simulink model "adm_pcie_9h7_dts_dual_4x100g_dts_test"  (R2019a)
settings: Solver=VariableStepAuto  StartTime=0.0  StopTime=10.0  RelTol=1e-3
undefined symbols (not defined in the file or in its folder): datetime, posixtime
libraries: xbsIndex_r4 x4914, casper_library_misc x38, xps_library x11
(part 1 of 58)
settings Model: ModifiedComment=jackh -- Wed Aug 24 09:07:48 2022 -- Version 1.233  Creator=jackh  LastModifiedBy=jackh
settings Model: ModifiedHistory=|
  | jackh -- Wed Aug 24 09:07:48 2022 -- Version 1.233
  | 
  | jackh -- Tue Aug 23 10:15:12 2022 -- Version 1.232
  | 
  | jackh -- Tue Aug 23 10:08:31 2022 -- Version 1.231
  | 
  | jackh -- Thu Aug 18 20:38:32 2022 -- Version 1.230
  | 
  | v13.4 bugfix 1
  | Rebuild with DTS buffer fixes
  | 
  | jackh -- Thu Aug 04 11:53:58 2022 -- Version 1.229
  | 
  | as compiled
  | 
  | jackh -- Wed Aug 03 18:39:00 2022 -- Version 1.228
  | 
  | v13.4 -- add post quant TVG which is a counter with spectrum number
  | 
  | jackh -- Wed Aug 03 12:22:54 2022 -- Version 1.227
  | 
  | as compiled
  | 
  | jackh -- Tue Aug 02 16:59:19 2022 -- Version 1.226
  | 
  | v13.3.3
  | 
  | Make LO offset input accept signed values
  | 
  | jackh -- Thu Jul 14 12:25:27 2022 -- Version 1.225
  | v13.3.2
  | 
  | change sine/cos lookup tables to 18-bit depth
  | 
  | jackh -- Fri Jul 08 12:09:48 2022 -- Version 1.224
  | 
  | jackh -- Fri Jul 08 11:59:21 2022 -- Version 1.223
  | 
  | 13.3.1
  | 
  | Make LO shift phase register 32_29
  | 
  | jackh -- Tue Jul 05 14:22:39 2022 -- Version 1.222
  | 
  | 13.2.4
  | 
  | Add 100G output snapshots and stats counters
  | 
  | jackh -- Fri Jun 17 09:21:46 2022 -- Version 1.221
  | 
  | Make PR template file relative. Increment fw revision
  | 
  | jackh -- Fri May 20 08:03:37 2022 -- Version 1.220
  | 
  | jackh -- Thu May 19 16:47:03 2022 -- Version 1.219
  | 
  | jackh -- Thu May 19 16:07:36 2022 -- Version 1.218
  | 
  | 13.2.2
  | 
  | Increase coarse delay to 512 samples
  | 
  | jackh -- Thu May 19 15:48:23 2022 -- Version 1.217
  | 
  | pipeline time offset
  | 
  | jackh -- Thu May 19 15:45:17 2022 -- Version 1.216
  | 
  | v13.2.1
  | 
  | Add aux time measurement
  | 
  | jackh -- Tue May 03 22:22:24 2022 -- Version 1.215
  | 
  | jackh -- Tue May 03 12:52:13 2022 -- Version 1.214
  | 
  | 13.2.0.1
  | 
  | - Fix FFT syncout period (now infinite)
  | - Add max_delay register to delay subsystem
  | 
  | jackh -- Tue May 03 11:06:51 2022 -- Version 1.213
  | 
  | v13.2 (should have been 13) as compiled
  | 
  | jackh -- Mon May 02 12:19:53 2022 -- Version 1.212
  | 
  | jackh -- Mon May 02 12:13:43 2022 -- Version 1.211
  | 
  | jackh -- Mon May 02 12:03:22 2022 -- Version 1.210
  | 
  | Move to 1MHz channels (2048-chan PFB; 1024 sent chans)
  | Incorporate FFT descramble mlib_devel fix
  | 
  | jackh -- Thu Apr 07 10:41:20 2022 -- Version 1.209
  | 
  | compiled
  | 
  | jackh -- Wed Apr 06 17:17:38 2022 -- Version 1.208
  | 
  | Bugfix 1
  | 
  | - Change LO offset so real part os cosine mixer (so mixing with DC does nothing)
  | - Fix cross-corr conjugation
  | - Fix cross corr acc_len computation
  | 
  | jackh -- Thu Mar 24 11:16:10 2022 -- Version 1.207
  | 
  | jackh -- Wed Mar 23 15:55:29 2022 -- Version 1.206
  | 
  | v12.2 Add sine wave generators to both pipelines.
  | Default to no added sine wave.
  | 
  | jackh -- Wed Mar 23 15:38:55 2022 -- Version 1.205
  | 
  | jackh -- Wed Mar 23 15:24:07 2022 -- Version 1.204
  | 
  | delay match sine generation and data streams
  | 
  | jackh -- Wed Mar 23 15:22:28 2022 -- Version 1.203
  | 
  | jackh -- Wed Mar 23 15:14:26 2022 -- Version 1.202
  | 
  | Add additive sinewave TVG
  | 
  | jackh -- Wed Mar 23 15:12:01 2022 -- Version 1.201
  | 
  | jackh -- Tue Mar 08 10:23:22 2022 -- Version 1.200
  | 
  | jackh -- Mon Mar 07 17:18:28 2022 -- Version 1.199
  | 
  | jackh -- Mon Mar 07 17:10:55 2022 -- Version 1.198
  | 
  | jackh -- Mon Mar 07 16:45:17 2022 -- Version 1.197
  | 
  | jackh -- Mon Mar 07 16:37:10 2022 -- Version 1.196
  | 
  | Add Corr block.
  | Allows examination of post-quantization signals, and
  | to cross correlate different IFs (useful for testing
  | in internal noisegen mode)
  | 
  | jackh -- Mon Mar 07 16:13:50 2022 -- Version 1.195
  | 
  | PFB band select reorder depth fix
  | 
  | jackh -- Thu Mar 03 13:08:01 2022 -- Version 1.194
  | 
  | jackh -- Tue Mar 01 20:34:16 2022 -- Version 1.193
  | 
  | jackh -- Tue Mar 01 17:19:43 2022 -- Version 1.192
  | 
  | jackh -- Tue Mar 01 17:10:04 2022 -- Version 1.191
  | 
  | jackh -- Tue Mar 01 16:55:54 2022 -- Version 1.190
  | 
  | jackh -- Tue Mar 01 16:45:57 2022 -- Version 1.189
  | 
  | jackh -- Tue Mar 01 15:57:56 2022 -- Version 1.188
  | 
  | jackh -- Tue Mar 01 15:49:45 2022 -- Version 1.187
  | 
  | jackh -- Tue Mar 01 15:22:14 2022 -- Version 1.186
  | 
  | jackh -- Mon Feb 28 13:26:19 2022 -- Version 1.185
  | 
  | jackh -- Mon Feb 28 13:08:19 2022 -- Version 1.184
  | 
  | jackh -- Sat Feb 26 14:41:54 2022 -- Version 1.183
  | 
  | jackh -- Fri Feb 25 18:46:11 2022 -- Version 1.182
  | 
  | jackh -- Fri Feb 25 18:45:03 2022 -- Version 1.181
  | 
  | jackh -- Thu Feb 24 15:51:36 2022 -- Version 1.180
  | 
  | update noisegen casting (just take MSBs)
  | 
  | jackh -- Thu Feb 24 15:08:58 2022 -- Version 1.179
  | 
  | v12
  | 
  | jackh -- Thu Feb 24 15:06:46 2022 -- Version 1.178
  | 
  | Move to 4x100G template
  | 
  | 
  | jackh -- Thu Feb 24 15:02:10 2022 -- Version 1.177
  | 
  | jackh -- Wed Feb 09 19:02:50 2022 -- Version 1.176
  | 
  | jackh -- Wed Feb 09 10:59:16 2022 -- Version 1.175
  | 
  | Try _again_ to fix timestamp issue.
  | This time the fix was actually simulated, and seems to work.
  | 
  | jackh -- Wed Feb 09 10:58:22 2022 -- Version 1.174
  | 
  | jackh -- Wed Feb 09 10:34:47 2022 -- Version 1.173
  | 
  | jackh -- Tue Feb 08 22:13:18 2022 -- Version 1.172
  | 
  | Change autocorr pipelining to fix timing errors
  | 
  | jackh -- Tue Feb 08 11:22:49 2022 -- Version 1.171
  | 
  | Try (again) to fix MCNT offset issue.
  | This time just propagate the time_step_bit lower MCNT counter
  | bits through to the header.
  | 
  | jackh -- Tue Feb 08 08:36:48 2022 -- Version 1.170
  | 
  | jackh -- Mon Feb 07 16:56:49 2022 -- Version 1.169
  | 
  | jackh -- Mon Feb 07 16:34:15 2022 -- Version 1.168
  | 
  | jackh -- Mon Feb 07 16:26:49 2022 -- Version 1.167
  | 
  | jackh -- Mon Feb 07 12:47:03 2022 -- Version 1.166
  | 
  | jackh -- Mon Feb 07 12:32:35 2022 -- Version 1.165
  | 
  | Add TT sync register, storing the time of the last sync
  | 
  | jackh -- Mon Feb 07 12:23:30 2022 -- Version 1.164
  | 
  | increment bugfix to 11.0.0.2
  | 
  | 
  | jackh -- Mon Feb 07 12:22:16 2022 -- Version 1.163
  | 
  | Propagate LSBs of sync time to packet headers
  | 
  | jackh -- Sat Feb 05 22:32:38 2022 -- Version 1.162
  | 
  | jackh -- Sat Feb 05 18:43:37 2022 -- Version 1.161
  | 
  | v11
  | More changes to reorder.
  | Process ADC data at 8 (not 12) bit resolution
  | Use URAM via black-box imports for coarse delay and big channel reorder
  | 
  | jackh -- Sat Feb 05 18:36:04 2022 -- Version 1.160
  | 
  | jackh -- Sat Feb 05 17:38:40 2022 -- Version 1.159
  | 
  | jackh -- Sat Feb 05 17:24:29 2022 -- Version 1.158
  | 
  | jackh -- Sat Feb 05 17:22:21 2022 -- Version 1.157
  | 
  | jackh -- Fri Feb 04 17:40:07 2022 -- Version 1.156
  | 
  | jackh -- Fri Feb 04 12:37:39 2022 -- Version 1.155
  | 
  | 64 times per packet
  | 
  | 
  | jackh -- Thu Feb 03 21:55:46 2022 -- Version 1.154
  | 
  | as compiled
  | 
  | 
  | jackh -- Thu Feb 03 14:45:04 2022 -- Version 1.153
  | 
  | jackh -- Thu Feb 03 14:28:02 2022 -- Version 1.152
  | 
  | jackh -- Thu Feb 03 13:59:18 2022 -- Version 1.151
  | 
  | jackh -- Thu Feb 03 11:15:21 2022 -- Version 1.150
  | 
  | jackh -- Wed Feb 02 16:47:47 2022 -- Version 1.149
  | 
  | jackh -- Wed Feb 02 16:40:11 2022 -- Version 1.148
  | 
  | Fix incorrect final transpose in reorder block
  | 
  | jackh -- Wed Feb 02 16:16:13 2022 -- Version 1.147
  | 
  | v8. Add channel reordering
  | 
  | Not actually necessary for 8-bit mode, but will
  | facilitate testing which is necessary for 3-bit mode
  | 
  | jackh -- Wed Feb 02 10:37:50 2022 -- Version 1.146
  | 
  | 7.0.1
  | 
  | Change coarse delay bram latency to 3 (hopefully will fix small timing fail)
  | 
  | jackh -- Wed Feb 02 10:34:03 2022 -- Version 1.145
  | 
  | jackh -- Tue Feb 01 14:52:02 2022 -- Version 1.144
  | 
  | Don't use ultraRAM for coarse delay (but we should!)
  | because it breaks sysgen. Sigh.
  | 
  | jackh -- Tue Feb 01 14:27:12 2022 -- Version 1.143
  | 
  | jackh -- Tue Feb 01 14:18:24 2022 -- Version 1.142
  | 
  | v7. Add noisegen / coarse delay
  | 
  | jackh -- Tue Feb 01 14:12:26 2022 -- Version 1.141
  | 
  | jackh -- Tue Feb 01 14:09:37 2022 -- Version 1.140
  | 
  | jackh -- Tue Feb 01 11:46:40 2022 -- Version 1.139
  | 
  | jackh -- Tue Feb 01 11:12:13 2022 -- Version 1.138
  | 
  | Add noise gen
  | 
  | jackh -- Tue Feb 01 11:01:17 2022 -- Version 1.137
  | 
  | v6.1 Harmonize input ordering convention by flipping
  | inputs so "input 0" is MSBs of data
  | 
  | jackh -- Tue Feb 01 10:38:57 2022 -- Version 1.136
  | 
  | jackh -- Mon Jan 31 13:11:04 2022 -- Version 1.135
  | 
  | jackh -- Mon Jan 31 12:33:38 2022 -- Version 1.134
  | 
  | jackh -- Mon Jan 31 12:25:15 2022 -- Version 1.133
  | 
  | jackh -- Fri Jan 28 17:22:49 2022 -- Version 1.132
  | 
  | jackh -- Fri Jan 28 17:16:19 2022 -- Version 1.131
  | 
  | jackh -- Fri Jan 28 17:06:25 2022 -- Version 1.130
  | 
  | v6.0 Add input bitstats / simulation mux
  | 
  | jackh -- Fri Jan 28 17:02:52 2022 -- Version 1.129
  | 
  | jackh -- Fri Jan 28 16:59:39 2022 -- Version 1.128
  | 
  | jackh -- Fri Jan 28 16:55:40 2022 -- Version 1.127
  | 
  | jackh -- Fri Jan 28 16:17:24 2022 -- Version 1.126
  | 
  | v5.0.2 Fix potential (but unliekly) issue with sync arm coinciding
  | with sync pulse
  | 
  | 
  | jackh -- Fri Jan 28 16:01:17 2022 -- Version 1.125
  | 
  | Attempt to fix DTS alignment unreliability (control signal CDC issue in mlib_devel)
  | 
  | jackh -- Fri Jan 28 12:51:42 2022 -- Version 1.124
  | 
  | as compiled
  | 
  | jackh -- Thu Jan 27 16:47:33 2022 -- Version 1.123
  | 
  | v5.0
  | 
  | Add sync gen logic
  | 
  | jackh -- Thu Jan 27 11:25:49 2022 -- Version 1.122
  | 
  | v4.1 Add index interval error counter
  | 
  | jackh -- Thu Jan 27 11:22:02 2022 -- Version 1.121
  | 
  | Make index 50ms -- add not-locked counter
  | 
  | 
  | jackh -- Thu Jan 27 10:32:00 2022 -- Version 1.120
  | 
  | Recompile using raw "index" pulse. Add index snapshots
  | 
  | jackh -- Wed Jan 26 15:06:47 2022 -- Version 1.119
  | 
  | jackh -- Wed Jan 26 13:46:28 2022 -- Version 1.118
  | 
  | jackh -- Wed Jan 26 13:04:56 2022 -- Version 1.117
  | 
  | jackh -- Tue Jan 25 18:32:15 2022 -- Version 1.116
  | 
  | Add index (10ms pulse?) count logic
  | 
  | jackh -- Tue Jan 25 18:31:36 2022 -- Version 1.115
  | 
  | jackh -- Tue Jan 25 11:48:12 2022 -- Version 1.114
  | 
  | jackh -- Tue Jan 25 11:41:44 2022 -- Version 1.113
  | 
  | jackh -- Tue Jan 25 11:38:37 2022 -- Version 1.112
  | 
  | Readd autocorr (needed behavioural complex mults)
  | 
  | jackh -- Mon Jan 24 20:49:54 2022 -- Version 1.111
  | 
  | comment out autocorr (causing compile fails)
  | 
  | jackh -- Mon Jan 24 20:10:36 2022 -- Version 1.110
  | 
  | jackh -- Mon Jan 24 19:58:33 2022 -- Version 1.109
  | 
  | jackh -- Mon Jan 24 19:53:28 2022 -- Version 1.108
  | 
  | autocorr floating point error fixes
  | 
  | 
  | jackh -- Mon Jan 24 19:51:34 2022 -- Version 1.107
  | 
  | jackh -- Mon Jan 24 18:28:31 2022 -- Version 1.106
  | 
  | jackh -- Mon Jan 24 18:27:12 2022 -- Version 1.105
  | 
  | Add autocorr (to pipeline 0)
  | 
  | jackh -- Mon Jan 24 18:15:24 2022 -- Version 1.104
  | 
  | Add EQTVG
  | 
  | jackh -- Mon Jan 24 13:19:54 2022 -- Version 1.103
settings DataIOCC: ReturnWorkspaceOutputs=off
settings DebuggingCC: PregeneratedLibrarySubsystemCodeDiagnostic=none  ArithmeticOperatorsInVariantConditions=warning
settings SFSimCC: SimUseLocalCustomCode=off
settings RTWCC: RTWUseLocalCustomCode=off

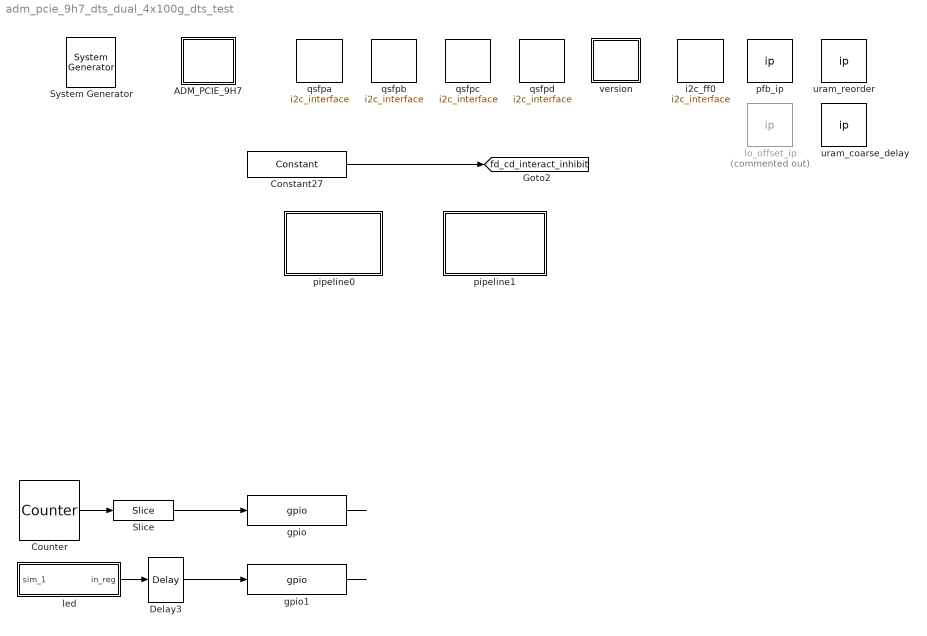
== system adm_pcie_9h7_dts_dual_4x100g_dts_test ==
  " System Generator" : xbsIndex_r4/ System Generator  Tag=genX  xilinxfamily=virtexuplusHBM  part=xcvu37p  speed=-2-e  package=fsvh2892  synthesis_tool=XST  clock_wrapper=Clock Enables  directory=/home/jackh/src/vla-dev/firmware/adm_pcie_9h7_dts_dual_4x100g_dts_test/sysgen  proj_type=Vivado  Synth_file=Vivado Synthesis Defaults  Impl_file=Vivado Implementation Defaults  testbench=off  simulink_period=1  sysclk_period=3.9062  dcm_input_clock_period=10  incr_netlist=off  trim_vbits=Everywhere in SubSystem  dbl_ovrd=According to Block Masks  core_generation=According to Block Masks  run_coregen=off  deprecated_control=off  eval_field=0  block_type=sysgen
  ADM_PCIE_9H7 : Subsystem  Tag=xps:xsg  mask(xsg core config){hw_sys=ADM_PCIE_9H7:xcvu37p, clk_src=dts_clk, clk_rate=256, use_microblaze=off, use_pr=on, pr_template=[fileparts(which(bdroot)) '/pr_templates/adm_pcie_9h7_dts_dual_4x100g_pr_template-no-ip.xpr.zip'], sample_period=1, synthesis_tool=XST}
      mask prompts: hw_sys "Hardware Platform"; clk_src "User IP Clock source"; clk_rate "User IP Clock Rate (MHz)"; use_microblaze "Use Microblaze controller?"; use_pr "Use PCIe Partial Reconfiguration"; sample_period "Sample Period"; synthesis_tool "Synthesis Tool:"
      mask help:
      | The XSG Core Config block is used to configure the System Generator design
      | for the casper_xps toolflow. Settings here are used to configure the
      | Xilinx System Generator block parameters automatically, and control toolflow
      | script  execution. It needs to be at the top level of all designs being compiled
      | with the casper_xps toolflow.
      mask init:
      | xps_xsg_adm_pcie_9h7_conf_mask;
      mask Help: eval('xlWeb([getenv(''MLIB_ROOT''), ''\doc\html\sys_xsg_core_config\sys_xsg_core_config.html''])')
      mask TypeOptions hw_sys: ADM_PCIE_9H7:xcvu37p
      mask TypeOptions clk_src: sys_clk | dts_clk
      mask TypeOptions synthesis_tool: Leonardo Spectrum | Synplify | Synplify Pro | XST
      mask Display: fprintf(['ADM\nPCIE_9H7']);
  Constant27 : xbsIndex_r4/Constant  const=1  gui_display_data_type=Boolean  arith_type=Boolean  n_bits=32  bin_pt=31  preci_type=Single  exp_width=8  frac_width=24  explicit_period=on  period=1  equ=P=C  opselect=C  inp2=PCIN>>17  opr=+  inp1=P  carry=CIN  dbl_ovrd=off  block_type=constant
  Counter : xbsIndex_r4/Counter  cnt_type=Free Running  cnt_to=Inf  operation=Up  start_count=0  cnt_by_val=1  arith_type=Unsigned  n_bits=27  bin_pt=0  load_pin=off  rst=off  en=off  explicit_period=on  period=1  use_behavioral_HDL=off  implementation=Fabric  dbl_ovrd=off  block_type=counter
  Delay3 : xbsIndex_r4/Delay  rst=off  infoeditControl=Selection of Reset will increase slice count due to use of real FFs and instead of SRLs  en=off  latency=1  reg_retiming=off  dbl_ovrd=off  block_type=delay
  Slice : xbsIndex_r4/Slice  nbits=2  boolean_output=off  mode=Upper Bit Location + Width  bit1=0  base1=MSB of Input  bit0=0  base0=LSB of Input  dbl_ovrd=off  block_type=slice
  gpio : xps_library/IO/gpio  Tag=xps:gpio  io_group_params_forwarded=off  io_group=ROACH:led  io_group_real=led  io_group_custom=0  io_dir=out  arith_type=Unsigned  bitwidth=2  bin_pt=0  bit_index=[0 1]  sample_period=1  use_single_ended=off  use_ddr=off  reg_iob=on  reg_clk_phase=0  termination=None
      settings: SourceProductName=CASPER XPS Blockset
  gpio1 : xps_library/IO/gpio  Tag=xps:gpio  io_group_params_forwarded=off  io_group=ROACH:led  io_group_real=led  io_group_custom=0  io_dir=out  arith_type=Boolean  bitwidth=1  bin_pt=0  bit_index=2  sample_period=1  use_single_ended=off  use_ddr=off  reg_iob=on  reg_clk_phase=0  termination=None
      settings: SourceProductName=CASPER XPS Blockset
  i2c_ff0 : xps_library/IO/i2c_interface  Tag=xps:i2c_interface  sda_gpio='gpio'  sda_gpio_index=8  scl_gpio='gpio'  scl_gpio_index=7
      settings: SourceProductName=CASPER XPS Blockset
  led : Subsystem  Tag=xps:sw_reg  AncestorBlock=xps_library/Memory/software_register  mask(swreg){io_dir=From Processor, io_delay=0, init_val=0, sample_period=1, names=reg, bitwidths=1, bin_pts=0, arith_types=2, sim_port=on, show_format=on}
      mask prompts: io_dir "I/O direction"; io_delay "I/O delay"; init_val "Initial Value"; sample_period "Sample period"; names "Bitfield names [msb...lsb]"; bitwidths "Bitfield widths"; bin_pts "Bitfield binary pts"; arith_types "Bitfield types, ufix=0, fix=1, bool=2"; sim_port "Provide sim input/output?"; show_format "Print format string?"
      mask help: A 32-bit software-accessible register. Can be divided into bitfields of varying widths and types using the fields in the block mask.
      mask init:
      | swreg_init(gcb)
      settings: AttributesFormatString=1input:b = 1 bits
      mask TypeOptions io_dir: To Processor | From Processor
      mask Callback io_dir:
      | mask_enables = get_param(gcb, 'MaskEnables');
      | mask_names = get_param(gcb, 'MaskNames');
      | if strcmp(get_param(gcb, 'io_dir'), 'To Processor'),
      |     mask_enables{ismember(mask_names, 'sample_period')} = 'off';
      | else
      |     mask_enables{ismember(mask_names, 'sample_period')} = 'on';
      | end
      | set_param(gcb, 'MaskEnables', mask_enables);
      mask DialogControl ParameterTabVar0 Prompt: Setup
  lo_offset_ip : xps_library/Utilities/ip  Tag=xps:ip  Commented=on  lib_path=[fileparts(which(bdroot)) '/dsp/mixer_dec_8x_8i_8o_core']  ip_name='mixer_dec_8x_8i_8o_core'
      settings: SourceProductName=CASPER XPS Blockset
  pfb_ip : xps_library/Utilities/ip  Tag=xps:ip  lib_path=[fileparts(which(bdroot)) '/dsp/pfb_cplx_2p_2048c_16i_18o_core']  ip_name='pfb_cplx_2p_2048c_16i_18o_core'
      settings: SourceProductName=CASPER XPS Blockset
  pipeline0 : Subsystem
  pipeline1 : Subsystem
  qsfpa : xps_library/IO/i2c_interface  Tag=xps:i2c_interface  sda_gpio='qsfp_sda'  sda_gpio_index=0  scl_gpio='qsfp_scl'  scl_gpio_index=0
      settings: SourceProductName=CASPER XPS Blockset
  qsfpb : xps_library/IO/i2c_interface  Tag=xps:i2c_interface  sda_gpio='qsfp_sda'  sda_gpio_index=1  scl_gpio='qsfp_scl'  scl_gpio_index=1
      settings: SourceProductName=CASPER XPS Blockset
  qsfpc : xps_library/IO/i2c_interface  Tag=xps:i2c_interface  sda_gpio='qsfp_sda'  sda_gpio_index=2  scl_gpio='qsfp_scl'  scl_gpio_index=2
      settings: SourceProductName=CASPER XPS Blockset
  qsfpd : xps_library/IO/i2c_interface  Tag=xps:i2c_interface  sda_gpio='qsfp_sda'  sda_gpio_index=3  scl_gpio='qsfp_scl'  scl_gpio_index=3
      settings: SourceProductName=CASPER XPS Blockset
  uram_coarse_delay : xps_library/Utilities/ip  Tag=xps:ip  lib_path=[fileparts(which(bdroot)) '/dsp/uram_dp_64kx64_latency3_core']  ip_name='uram_dp_64kx64_latency3_core'
      settings: SourceProductName=CASPER XPS Blockset
  uram_reorder : xps_library/Utilities/ip  Tag=xps:ip  lib_path=[fileparts(which(bdroot)) '/dsp/uram_8192x512_latency3_core']  ip_name='uram_8192x512_latency3_core'
      settings: SourceProductName=CASPER XPS Blockset
  version : Subsystem  mask{fw_type=99, ver_maj=1, ver_min=0, ver_rev=0, ver_bugfix=0}
      mask prompts: fw_type "Firmware Type"; ver_maj "Major version"; ver_min "Minor version"; ver_rev "Revision"; ver_bugfix "Bugfix"
  tag scope: fd_cd_interact_inhibit=global
  wires:
  gpio/1 -> ?
  Delay3/1 -> gpio1/1
  Counter/1 -> Slice/1
  gpio1/1 -> ?
  led/1(in_reg) -> Delay3/1
  Slice/1 -> gpio/1
  Constant27/1 -> [fd_cd_interact_inhibit]

== system adm_pcie_9h7_dts_dual_4x100g_dts_test/ADM_PCIE_9H7 ==

== system adm_pcie_9h7_dts_dual_4x100g_dts_test/led ==
  sim_1 : Inport
  adm_pcie_9h7_dts_dual_4x100g_dts_test_led_user_data_out : xbsIndex_r4/Gateway In  gui_display_data_type=Fixed-point  arith_type=Unsigned  n_bits=32  bin_pt=0  preci_type=Single  exp_width=8  frac_width=24  rows=1  columns=1  quantization="Round  (unbiased: +/- Inf)"  overflow=Saturate  period=1  UseAsADC=off  ADCChannel='1'  interface=None  automatic_assignment=on  address_offset=hex2dec('00')  intf_name=''  intf_description=''  default_value=0  timing_constraint=None  locs_specified=off  LOCs={}  io_standard={}  inherit_from_input=off  hdl_port=on  dbl_ovrd=off  block_type=gatewayin
  convert1_1 : DataTypeConversion  OutDataTypeStr=fixdt('ufix1_En0')  LockScale=on
  convert2_1 : DataTypeConversion  OutDataTypeStr=fixdt('ufix1_En0')  ConvertRealWorld=Stored Integer (SI)  LockScale=on
  gain_1 : Gain
  io_delay : xbsIndex_r4/Delay  rst=off  infoeditControl=Selection of Reset will increase slice count due to use of real FFs and instead of SRLs  en=off  latency=0  reg_retiming=on  dbl_ovrd=off  block_type=delay
  slice_reg : xbsIndex_r4/Slice  nbits=1  boolean_output=on  mode=Lower Bit Location + Width  bit1=0  base1=MSB of Input  bit0=0  base0=LSB of Input  dbl_ovrd=off  block_type=slice
  in_reg : Outport
  wires:
  adm_pcie_9h7_dts_dual_4x100g_dts_test_led_user_data_out/1 -> io_delay/1
  sim_1/1 -> convert1_1/1
  convert1_1/1 -> convert2_1/1
  convert2_1/1 -> gain_1/1
  gain_1/1 -> adm_pcie_9h7_dts_dual_4x100g_dts_test_led_user_data_out/1
  io_delay/1 -> slice_reg/1
  slice_reg/1 -> in_reg/1

== system adm_pcie_9h7_dts_dual_4x100g_dts_test/pipeline0 ==
  note: 4 inputs (2 IFs x dual pol)
      |
      | Each 8 parallel words x 12 bits
      | (96 bits per input)
      | (384 bits total)
  Constant : xbsIndex_r4/Constant  const=0  gui_display_data_type=Fixed-point  arith_type=Unsigned  n_bits=64  bin_pt=0  preci_type=Single  exp_width=8  frac_width=24  explicit_period=on  period=1  equ=P=C  opselect=C  inp2=PCIN>>17  opr=+  inp1=P  carry=CIN  dbl_ovrd=off  block_type=constant
  Constant1 : xbsIndex_r4/Constant  const=0  gui_display_data_type=Fixed-point  arith_type=Unsigned  n_bits=16  bin_pt=0  preci_type=Single  exp_width=8  frac_width=24  explicit_period=on  period=1  equ=P=C  opselect=C  inp2=PCIN>>17  opr=+  inp1=P  carry=CIN  dbl_ovrd=off  block_type=constant
  Constant{3..4,9..10} (4 alike) : xbsIndex_r4/Constant  const=0  gui_display_data_type=Boolean  arith_type=Boolean  n_bits=32  bin_pt=0  preci_type=Single  exp_width=8  frac_width=24  explicit_period=on  period=1  equ=P=C  opselect=C  inp2=PCIN>>17  opr=+  inp1=P  carry=CIN  dbl_ovrd=off  block_type=constant
  Constant11 : xbsIndex_r4/Constant  const=0  gui_display_data_type=Fixed-point  arith_type=Unsigned  n_bits=512  bin_pt=0  preci_type=Single  exp_width=8  frac_width=24  explicit_period=on  period=1  equ=P=C  opselect=C  inp2=PCIN>>17  opr=+  inp1=P  carry=CIN  dbl_ovrd=off  block_type=constant
  Constant2 : xbsIndex_r4/Constant  const=0  gui_display_data_type=Fixed-point  arith_type=Unsigned  n_bits=32  bin_pt=0  preci_type=Single  exp_width=8  frac_width=24  explicit_period=on  period=1  equ=P=C  opselect=C  inp2=PCIN>>17  opr=+  inp1=P  carry=CIN  dbl_ovrd=off  block_type=constant
  Constant5 : xbsIndex_r4/Constant  const=0  gui_display_data_type=Fixed-point  arith_type=Unsigned  n_bits=512  bin_pt=0  preci_type=Single  exp_width=8  frac_width=24  explicit_period=on  period=1  equ=P=C  opselect=C  inp2=PCIN>>17  opr=+  inp1=P  carry=CIN  dbl_ovrd=off  block_type=constant
  Constant6 : xbsIndex_r4/Constant  const=0  gui_display_data_type=Fixed-point  arith_type=Unsigned  n_bits=64  bin_pt=0  preci_type=Single  exp_width=8  frac_width=24  explicit_period=on  period=1  equ=P=C  opselect=C  inp2=PCIN>>17  opr=+  inp1=P  carry=CIN  dbl_ovrd=off  block_type=constant
  Constant7 : xbsIndex_r4/Constant  const=0  gui_display_data_type=Fixed-point  arith_type=Unsigned  n_bits=16  bin_pt=0  preci_type=Single  exp_width=8  frac_width=24  explicit_period=on  period=1  equ=P=C  opselect=C  inp2=PCIN>>17  opr=+  inp1=P  carry=CIN  dbl_ovrd=off  block_type=constant
  Constant8 : xbsIndex_r4/Constant  const=0  gui_display_data_type=Fixed-point  arith_type=Unsigned  n_bits=32  bin_pt=0  preci_type=Single  exp_width=8  frac_width=24  explicit_period=on  period=1  equ=P=C  opselect=C  inp2=PCIN>>17  opr=+  inp1=P  carry=CIN  dbl_ovrd=off  block_type=constant
  dts : Subsystem
  eth0 : Subsystem
  eth1 : Subsystem
  wires:
  dts/2(dout) -> ?
  Constant/1 -> eth1/6(byte_enable)
  Constant1/1 -> eth1/5(dest_port)
  Constant2/1 -> eth1/4(dest_ip)
  Constant5/1 -> eth1/1(data)
  Constant4/1 -> eth1/2(vld)
  Constant3/1 -> eth1/3(eof)
  Constant9/1 -> eth0/3(eof)
  Constant10/1 -> eth0/2(vld)
  Constant11/1 -> eth0/1(data)
  Constant8/1 -> eth0/4(dest_ip)
  Constant7/1 -> eth0/5(dest_port)
  Constant6/1 -> eth0/6(byte_enable)

== system adm_pcie_9h7_dts_dual_4x100g_dts_test/pipeline1 ==
  note: 4 inputs (2 IFs x dual pol)
      |
      | Each 8 parallel words x 12 bits
      | (96 bits per input)
      | (384 bits total)
  Constant : xbsIndex_r4/Constant  const=0  gui_display_data_type=Fixed-point  arith_type=Unsigned  n_bits=64  bin_pt=0  preci_type=Single  exp_width=8  frac_width=24  explicit_period=on  period=1  equ=P=C  opselect=C  inp2=PCIN>>17  opr=+  inp1=P  carry=CIN  dbl_ovrd=off  block_type=constant
  Constant1 : xbsIndex_r4/Constant  const=0  gui_display_data_type=Fixed-point  arith_type=Unsigned  n_bits=16  bin_pt=0  preci_type=Single  exp_width=8  frac_width=24  explicit_period=on  period=1  equ=P=C  opselect=C  inp2=PCIN>>17  opr=+  inp1=P  carry=CIN  dbl_ovrd=off  block_type=constant
  Constant{3..4,9..10} (4 alike) : xbsIndex_r4/Constant  const=0  gui_display_data_type=Boolean  arith_type=Boolean  n_bits=32  bin_pt=0  preci_type=Single  exp_width=8  frac_width=24  explicit_period=on  period=1  equ=P=C  opselect=C  inp2=PCIN>>17  opr=+  inp1=P  carry=CIN  dbl_ovrd=off  block_type=constant
  Constant11 : xbsIndex_r4/Constant  const=0  gui_display_data_type=Fixed-point  arith_type=Unsigned  n_bits=512  bin_pt=0  preci_type=Single  exp_width=8  frac_width=24  explicit_period=on  period=1  equ=P=C  opselect=C  inp2=PCIN>>17  opr=+  inp1=P  carry=CIN  dbl_ovrd=off  block_type=constant
  Constant2 : xbsIndex_r4/Constant  const=0  gui_display_data_type=Fixed-point  arith_type=Unsigned  n_bits=32  bin_pt=0  preci_type=Single  exp_width=8  frac_width=24  explicit_period=on  period=1  equ=P=C  opselect=C  inp2=PCIN>>17  opr=+  inp1=P  carry=CIN  dbl_ovrd=off  block_type=constant
  Constant5 : xbsIndex_r4/Constant  const=0  gui_display_data_type=Fixed-point  arith_type=Unsigned  n_bits=512  bin_pt=0  preci_type=Single  exp_width=8  frac_width=24  explicit_period=on  period=1  equ=P=C  opselect=C  inp2=PCIN>>17  opr=+  inp1=P  carry=CIN  dbl_ovrd=off  block_type=constant
  Constant6 : xbsIndex_r4/Constant  const=0  gui_display_data_type=Fixed-point  arith_type=Unsigned  n_bits=64  bin_pt=0  preci_type=Single  exp_width=8  frac_width=24  explicit_period=on  period=1  equ=P=C  opselect=C  inp2=PCIN>>17  opr=+  inp1=P  carry=CIN  dbl_ovrd=off  block_type=constant
  Constant7 : xbsIndex_r4/Constant  const=0  gui_display_data_type=Fixed-point  arith_type=Unsigned  n_bits=16  bin_pt=0  preci_type=Single  exp_width=8  frac_width=24  explicit_period=on  period=1  equ=P=C  opselect=C  inp2=PCIN>>17  opr=+  inp1=P  carry=CIN  dbl_ovrd=off  block_type=constant
  Constant8 : xbsIndex_r4/Constant  const=0  gui_display_data_type=Fixed-point  arith_type=Unsigned  n_bits=32  bin_pt=0  preci_type=Single  exp_width=8  frac_width=24  explicit_period=on  period=1  equ=P=C  opselect=C  inp2=PCIN>>17  opr=+  inp1=P  carry=CIN  dbl_ovrd=off  block_type=constant
  dts : Subsystem
  eth0 : Subsystem
  eth1 : Subsystem
  wires:
  Constant3/1 -> eth1/3(eof)
  Constant4/1 -> eth1/2(vld)
  Constant5/1 -> eth1/1(data)
  Constant2/1 -> eth1/4(dest_ip)
  Constant1/1 -> eth1/5(dest_port)
  Constant/1 -> eth1/6(byte_enable)
  Constant6/1 -> eth0/6(byte_enable)
  Constant7/1 -> eth0/5(dest_port)
  Constant8/1 -> eth0/4(dest_ip)
  Constant11/1 -> eth0/1(data)
  Constant10/1 -> eth0/2(vld)
  Constant9/1 -> eth0/3(eof)

== system adm_pcie_9h7_dts_dual_4x100g_dts_test/version ==
  Concat : xbsIndex_r4/Concat  num_inputs=4  dbl_ovrd=off  block_type=concat
  Constant : xbsIndex_r4/Constant  const=ver_maj  gui_display_data_type=Fixed-point  arith_type=Unsigned  n_bits=8  bin_pt=0  preci_type=Single  exp_width=8  frac_width=24  explicit_period=on  period=1  equ=P=C  opselect=C  inp2=PCIN>>17  opr=+  inp1=P  carry=CIN  dbl_ovrd=off  block_type=constant
  Constant1 : xbsIndex_r4/Constant  const=ver_min  gui_display_data_type=Fixed-point  arith_type=Unsigned  n_bits=8  bin_pt=0  preci_type=Single  exp_width=8  frac_width=24  explicit_period=on  period=1  equ=P=C  opselect=C  inp2=PCIN>>17  opr=+  inp1=P  carry=CIN  dbl_ovrd=off  block_type=constant
  Constant2 : xbsIndex_r4/Constant  const=ver_rev  gui_display_data_type=Fixed-point  arith_type=Unsigned  n_bits=8  bin_pt=0  preci_type=Single  exp_width=8  frac_width=24  explicit_period=on  period=1  equ=P=C  opselect=C  inp2=PCIN>>17  opr=+  inp1=P  carry=CIN  dbl_ovrd=off  block_type=constant
  Constant3 : xbsIndex_r4/Constant  const=ver_bugfix  gui_display_data_type=Fixed-point  arith_type=Unsigned  n_bits=8  bin_pt=0  preci_type=Single  exp_width=8  frac_width=24  explicit_period=on  period=1  equ=P=C  opselect=C  inp2=PCIN>>17  opr=+  inp1=P  carry=CIN  dbl_ovrd=off  block_type=constant
  Constant4 : xbsIndex_r4/Constant  const=fw_type  gui_display_data_type=Fixed-point  arith_type=Unsigned  n_bits=32  bin_pt=0  preci_type=Single  exp_width=8  frac_width=24  explicit_period=on  period=1  equ=P=C  opselect=C  inp2=PCIN>>17  opr=+  inp1=P  carry=CIN  dbl_ovrd=off  block_type=constant
  Terminator1 : Terminator
  Terminator2 : Terminator
  timestamp : Subsystem  Tag=xps:sw_reg  AncestorBlock=xps_library/Memory/software_register  mask(swreg){io_dir=To Processor, io_delay=0, init_val=0, sample_period=1, names=reg, bitwidths=32, bin_pts=0, arith_types=0, sim_port=on, show_format=off, desc_str=Unix timestamp, in integer seconds, when firmware was last compiled.}
      mask prompts: io_dir "I/O direction"; io_delay "I/O delay"; init_val "Initial Value"; sample_period "Sample period"; names "Bitfield names [msb...lsb]"; bitwidths "Bitfield widths"; bin_pts "Bitfield binary pts"; arith_types "Bitfield types, ufix=0, fix=1, bool=2"; sim_port "Provide sim input/output?"; show_format "Print format string?"; desc_str "Description"
      mask help: A 32-bit software-accessible register. Can be divided into bitfields of varying widths and types using the fields in the block mask.
      mask init:
      | swreg_init(gcb)
      settings: AttributesFormatString=1output
      mask TypeOptions io_dir: To Processor | From Processor
      mask Callback io_dir:
      | mask_enables = get_param(gcb, 'MaskEnables');
      | mask_names = get_param(gcb, 'MaskNames');
      | if strcmp(get_param(gcb, 'io_dir'), 'To Processor'),
      |     mask_enables{ismember(mask_names, 'sample_period')} = 'off';
      | else
      |     mask_enables{ismember(mask_names, 'sample_period')} = 'on';
      | end
      | set_param(gcb, 'MaskEnables', mask_enables);
      mask DialogControl ParameterTabVar0 Prompt: Setup
  type : Subsystem  Tag=xps:sw_reg  AncestorBlock=xps_library/Memory/software_register  mask(swreg){io_dir=To Processor, io_delay=0, init_val=0, sample_period=1, names=reg, bitwidths=32, bin_pts=0, arith_types=0, sim_port=on, show_format=off, desc_str=|}
      mask desc_str=|
      | Version register. Bits ``[31:24]``: major version. Bits
      | ``[23:16]``: minor version. Bits ``[15:8]``: revision.
      | Bits ``[7:0]``: buxfix.
      mask prompts: io_dir "I/O direction"; io_delay "I/O delay"; init_val "Initial Value"; sample_period "Sample period"; names "Bitfield names [msb...lsb]"; bitwidths "Bitfield widths"; bin_pts "Bitfield binary pts"; arith_types "Bitfield types, ufix=0, fix=1, bool=2"; sim_port "Provide sim input/output?"; show_format "Print format string?"; desc_str "Description"
      mask help: A 32-bit software-accessible register. Can be divided into bitfields of varying widths and types using the fields in the block mask.
      mask init:
      | swreg_init(gcb)
      settings: AttributesFormatString=1output
      mask TypeOptions io_dir: To Processor | From Processor
      mask Callback io_dir:
      | mask_enables = get_param(gcb, 'MaskEnables');
      | mask_names = get_param(gcb, 'MaskNames');
      | if strcmp(get_param(gcb, 'io_dir'), 'To Processor'),
      |     mask_enables{ismember(mask_names, 'sample_period')} = 'off';
      | else
      |     mask_enables{ismember(mask_names, 'sample_period')} = 'on';
      | end
      | set_param(gcb, 'MaskEnables', mask_enables);
      mask DialogControl ParameterTabVar0 Prompt: Setup
  unix_time : xbsIndex_r4/Constant  const=round(posixtime(datetime('now')))  gui_display_data_type=Fixed-point  arith_type=Unsigned  n_bits=32  bin_pt=0  preci_type=Single  exp_width=8  frac_width=24  explicit_period=on  period=1  equ=P=C  opselect=C  inp2=PCIN>>17  opr=+  inp1=P  carry=CIN  dbl_ovrd=off  block_type=constant
  version : Subsystem  Tag=xps:sw_reg  AncestorBlock=xps_library/Memory/software_register  mask(swreg){io_dir=To Processor, io_delay=0, init_val=0, sample_period=1, names=reg, bitwidths=32, bin_pts=0, arith_types=0, sim_port=on, show_format=off, desc_str=|}
      mask desc_str=|
      | Version register. Bits ``[31:24]``: major version. Bits
      | ``[23:16]``: minor version. Bits ``[15:8]``: revision.
      | Bits ``[7:0]``: buxfix.
      mask prompts: io_dir "I/O direction"; io_delay "I/O delay"; init_val "Initial Value"; sample_period "Sample period"; names "Bitfield names [msb...lsb]"; bitwidths "Bitfield widths"; bin_pts "Bitfield binary pts"; arith_types "Bitfield types, ufix=0, fix=1, bool=2"; sim_port "Provide sim input/output?"; show_format "Print format string?"; desc_str "Description"
      mask help: A 32-bit software-accessible register. Can be divided into bitfields of varying widths and types using the fields in the block mask.
      mask init:
      | swreg_init(gcb)
      settings: AttributesFormatString=1output
      mask TypeOptions io_dir: To Processor | From Processor
      mask Callback io_dir:
      | mask_enables = get_param(gcb, 'MaskEnables');
      | mask_names = get_param(gcb, 'MaskNames');
      | if strcmp(get_param(gcb, 'io_dir'), 'To Processor'),
      |     mask_enables{ismember(mask_names, 'sample_period')} = 'off';
      | else
      |     mask_enables{ismember(mask_names, 'sample_period')} = 'on';
      | end
      | set_param(gcb, 'MaskEnables', mask_enables);
      mask DialogControl ParameterTabVar0 Prompt: Setup
  tag scope: ver_maj=global
  wires:
  Constant1/1 -> Concat/2
  Concat/1 -> version/1(out_reg)
  Constant/1 -> [ver_maj], Concat/1
  version/1(sim_out_reg) -> Terminator1/1
  Constant2/1 -> Concat/3
  Constant3/1 -> Concat/4
  timestamp/1(sim_out_reg) -> Terminator2/1
  unix_time/1 -> timestamp/1(out_reg)
  Constant4/1 -> type/1(out_reg)

== system adm_pcie_9h7_dts_dual_4x100g_dts_test/pipeline0/dts ==
  Constant : xbsIndex_r4/Constant  const=2^12 - 1  gui_display_data_type=Fixed-point  arith_type=Unsigned  n_bits=12  bin_pt=0  preci_type=Single  exp_width=8  frac_width=24  explicit_period=on  period=1  equ=P=C  opselect=C  inp2=PCIN>>17  opr=+  inp1=P  carry=CIN  dbl_ovrd=off  block_type=constant
  Delay2 : xbsIndex_r4/Delay  rst=off  infoeditControl=Selection of Reset will increase slice count due to use of real FFs and instead of SRLs  en=off  latency=1  reg_retiming=off  dbl_ovrd=off  block_type=delay
  Relational : xbsIndex_r4/Relational  mode=a=b  op_type=Bool  en=off  latency=1  dbl_ovrd=off  block_type=relational
  dts : Subsystem  Tag=xps:vla_dts  mask(vla_dts){port=qsfp_a_b_c, is_master=on, mux_factor_bits=2}
      mask prompts: port "Which port(s)?"; is_master "Is clocking master (only set this for one DTS block)"; mux_factor_bits "Multiplex factor (2^?)"
      mask help: Receive VLA DTS data
      mask init:
      | vla_dts_mask(gcb)
      mask TypeOptions port: qsfp_a_b_c | firefly0 | firefly1
  edge_detect2 : casper_library_misc/edge_detect  edge=Rising  polarity=Active High  x_in=[0 0.08 0.08 0.16 0.16 0.24 0.24 0.32 0.32 0.4]  y_in="[-1 -1  1  1  1  1  1  1  1  1]"  x_out=[0.6 0.68 0.68 0.76 0.76 0.84 0.84 0.92 0.92 1]  y_out="[-1 -1  1  1 -1 -1 -1 -1 -1 -1]"
  flip_inputs : Subsystem
  rst : Subsystem  Tag=xps:sw_reg  AncestorBlock=xps_library/Memory/software_register  mask(swreg){io_dir=From Processor, io_delay=0, init_val=0, sample_period=1, names=reg, bitwidths=1, bin_pts=0, arith_types=2, sim_port=on, show_format=on}
      mask prompts: io_dir "I/O direction"; io_delay "I/O delay"; init_val "Initial Value"; sample_period "Sample period"; names "Bitfield names [msb...lsb]"; bitwidths "Bitfield widths"; bin_pts "Bitfield binary pts"; arith_types "Bitfield types, ufix=0, fix=1, bool=2"; sim_port "Provide sim input/output?"; show_format "Print format string?"
      mask help: A 32-bit software-accessible register. Can be divided into bitfields of varying widths and types using the fields in the block mask.
      mask init:
      | swreg_init(gcb)
      settings: AttributesFormatString=1input:b = 1 bits
      mask TypeOptions io_dir: To Processor | From Processor
      mask Callback io_dir:
      | mask_enables = get_param(gcb, 'MaskEnables');
      | mask_names = get_param(gcb, 'MaskNames');
      | if strcmp(get_param(gcb, 'io_dir'), 'To Processor'),
      |     mask_enables{ismember(mask_names, 'sample_period')} = 'off';
      | else
      |     mask_enables{ismember(mask_names, 'sample_period')} = 'on';
      | end
      | set_param(gcb, 'MaskEnables', mask_enables);
      mask DialogControl ParameterTabVar0 Prompt: Setup
  stats : Subsystem
  sync : Outport
  dout : Outport  Port=2
  wires:
  dts/4(ten_sec) -> stats/4(ten_sec)
  dts/5(locked) -> stats/5(lock)
  dts/6(sync) -> stats/6(sync)
  rst/1(in_reg) -> dts/1(rst)
  dts/3(one_sec) -> stats/3(pps)
  dts/2(index) -> Relational/1, stats/2(index)
  Delay2/1 -> dout/1
  Relational/1 -> edge_detect2/1
  edge_detect2/1 -> sync/1
  Constant/1 -> Relational/2
  flip_inputs/1(Out1) -> Delay2/1, stats/1(din)
  dts/1(frame_out) -> flip_inputs/1(In1)

== system adm_pcie_9h7_dts_dual_4x100g_dts_test/pipeline0/eth0 ==
  data : Inport
  vld : Inport  Port=2
  eof : Inport  Port=3
  dest_ip : Inport  Port=4
  dest_port : Inport  Port=5
  byte_enable : Inport  Port=6
  Constant : xbsIndex_r4/Constant  const=0  gui_display_data_type=Boolean  arith_type=Boolean  n_bits=1  bin_pt=0  preci_type=Single  exp_width=8  frac_width=24  explicit_period=on  period=1  equ=P=C  opselect=C  inp2=PCIN>>17  opr=+  inp1=P  carry=CIN  dbl_ovrd=off  block_type=constant
  Constant1 : xbsIndex_r4/Constant  const=0  gui_display_data_type=Boolean  arith_type=Boolean  n_bits=1  bin_pt=0  preci_type=Single  exp_width=8  frac_width=24  explicit_period=on  period=1  equ=P=C  opselect=C  inp2=PCIN>>17  opr=+  inp1=P  carry=CIN  dbl_ovrd=off  block_type=constant
  Delay : xbsIndex_r4/Delay  rst=off  infoeditControl=Selection of Reset will increase slice count due to use of real FFs and instead of SRLs  en=off  latency=1  reg_retiming=off  dbl_ovrd=off  block_type=delay
  Logical : xbsIndex_r4/Logical  logical_function=AND  inputs=2  en=off  latency=0  precision=Full  arith_type=Unsigned  n_bits=16  bin_pt=0  align_bp=on  dbl_ovrd=off  block_type=logical
  Register : xbsIndex_r4/Register  init=0  rst=off  en=on  dbl_ovrd=off  block_type=register
  Slice : xbsIndex_r4/Slice  nbits=1  boolean_output=on  mode=Lower Bit Location + Width  bit1=0  base1=MSB of Input  bit0=0  base0=LSB of Input  dbl_ovrd=off  block_type=slice
  Slice1 : xbsIndex_r4/Slice  nbits=1  boolean_output=on  mode=Lower Bit Location + Width  bit1=0  base1=MSB of Input  bit0=1  base0=LSB of Input  dbl_ovrd=off  block_type=slice
  Slice2 : xbsIndex_r4/Slice  nbits=16  boolean_output=off  mode=Lower Bit Location + Width  bit1=0  base1=MSB of Input  bit0=2  base0=LSB of Input  dbl_ovrd=off  block_type=slice
  Slice3 : xbsIndex_r4/Slice  nbits=1  boolean_output=on  mode=Lower Bit Location + Width  bit1=0  base1=MSB of Input  bit0=2+16  base0=LSB of Input  dbl_ovrd=off  block_type=slice
  ctrl : Subsystem  Tag=xps:sw_reg  AncestorBlock=xps_library/Memory/software_register  mask(swreg){io_dir=From Processor, io_delay=0, init_val=0, sample_period=1, names=reg, bitwidths=32, bin_pts=0, arith_types=0, sim_port=on, show_format=off}
      mask prompts: io_dir "I/O direction"; io_delay "I/O delay"; init_val "Initial Value"; sample_period "Sample period"; names "Bitfield names [msb...lsb]"; bitwidths "Bitfield widths"; bin_pts "Bitfield binary pts"; arith_types "Bitfield types, ufix=0, fix=1, bool=2"; sim_port "Provide sim input/output?"; show_format "Print format string?"
      mask help: A 32-bit software-accessible register. Can be divided into bitfields of varying widths and types using the fields in the block mask.
      mask init:
      | swreg_init(gcb)
      settings: AttributesFormatString=1input
      mask TypeOptions io_dir: To Processor | From Processor
      mask Callback io_dir:
      | mask_enables = get_param(gcb, 'MaskEnables');
      | mask_names = get_param(gcb, 'MaskNames');
      | if strcmp(get_param(gcb, 'io_dir'), 'To Processor'),
      |     mask_enables{ismember(mask_names, 'sample_period')} = 'off';
      | else
      |     mask_enables{ismember(mask_names, 'sample_period')} = 'on';
      | end
      | set_param(gcb, 'MaskEnables', mask_enables);
      mask DialogControl ParameterTabVar0 Prompt: Setup
  onehundred_gbe : Subsystem  Tag=xps:onehundred_gbe  AncestorBlock=xps_library/IO/onehundred_gbe  mask(forty_gbe){flavour=cx4, slot=1, port_r1=0, port_r2_cx4=0, port_r2_sfpp=0, port=3, rx_dist_ram=off, large_frames=on, input_pipeline_delay=0, show_param=off, pre_emph_r2=0.74, pre_emph=3, post_emph_r2=0.18, rxeqmix_r2=7, swing_r2=940, swing=800, fab_en=on, fab_mac=hex2dec('123456780000'), fab_ip=192*(2^24) + 168*(2^16) + 5*(2^8) + 20*(2^0), fab_udp=10000, fab_gate=1, cpu_rx_en=on, cpu_tx_en=on, ttl=hex2dec('FF'), promisc_mode=off, debug_ctr_width=32, debug_en_all=off, debug_dis_all=off, txctr=on, txerrctr=off, txerrctr_len=100, txofctr=on, txfullctr=on, txvldctr=on, txsnaplen=256, rxctr=off, rxerrctr=off, rxerrctr_len=100, rxofctr=off, rxbadctr=off, rxvldctr=off, rxeofctr=off, rxsnaplen=0 - no snap, rxsrcip=off, rxdstip=off}
      mask prompts: flavour "Mezzanine card flavour"; slot "Card slot"; port_r1 "Port"; port_r2_cx4 "Port"; port_r2_sfpp "Port"; rx_dist_ram "Shallow RX Fifo (Beware overruns!)"; large_frames "Enable Large TX Frames (8k+512)"; input_pipeline_delay "Incoming pipeline delay"; show_param "---------------------- Show Implementation Parameters -----------------------------------------------------------------------------------"; pre_emph_r2 "Pre-emphasis (dB)"; pre_emph "Pre-emphasis"; post_emph_r2 "Post-emphasis (dB)"; rxeqmix_r2 "Receive equalisation"; swing_r2 "Driver Swing Control (mVppd)"; swing "Differential swing"; fab_en "Enable fabric on startup"; fab_mac "Fabric MAC Address"; fab_ip "Fabric IP Address"; fab_udp "Fabric UDP Port"; fab_gate "Fabric Gateway"; cpu_rx_en "Enable CPU RX"; cpu_tx_en "Enable CPU TX"; promisc_mode "Promiscuous mode"; debug_ctr_width "Debug counter width"; debug_en_all "Enable all counters (overrides individual settings)"; debug_dis_all "Disable all counters (overrides individual settings)"; txctr "TX - core_txctr"; txerrctr "TX packet length error - core_txerrctr"; txerrctr_len "-- expected TX packet length"; txofctr "TX overflow - core_txofctr"; txfullctr "TX full - core_txfullctr"; txvldctr "TX valid cycle - core_txvldctr"; txsnaplen "TX snapshot length"; rxctr "RX - core_rxctr"; rxerrctr "RX packet length error - core_rxerrctr"; rxerrctr_len "-- expected RX packet length"; rxofctr "RX overflow - core_rxofctr"; rxbadctr "RX bad - core_rxbadctr"; rxvldctr "RX valid cycle - core_rxvldctr"; rxeofctr "RX eof - core_rxeofctr"; rxsnaplen "RX snapshot length"; rxsrcip "RX snapshot - include source IPs"; rxdstip "RX snapshot - include destination IPs"
      mask help: This block sends and receives UDP frames (packets). It accepts a 64 bit wide data stream with user-determined frame breaks. The data stream is wrapped in a UDP frame for transmission. Incoming UDP packets are unwrapped and the data presented as a 64 bit wide stream.
      mask init:
      | temp = eval(get_param(gcb, 'debug_ctr_width'));
      | if temp <= 0,
      |     error('Debug counters cannot be <= zero.');
      | end
      | onehundred_gbe_mask(gcb)
      settings: AttributesFormatString=incoming_latency=0
      mask TypeOptions flavour: sfp+ | cx4
      mask Callback flavour: forty_gbe_callback
      mask TypeOptions slot: 0 | 1
      mask TypeOptions port_r1: 0 | 1 | 2 | 3
      mask TypeOptions port_r2_cx4: 0 | 1 | 2
      mask TypeOptions port_r2_sfpp: 0 | 1 | 2 | 3
      mask Callback show_param: forty_gbe_callback
      mask TypeOptions pre_emph_r2: 0.15 | 0.3 | 0.45 | 0.61 | 0.74 | 0.91 | 1.07 | 1.25 | 1.36 | 1.55 | 1.74 | 1.94 | 2.11 | 2.32 | 2.54 | 2.77
      mask TypeOptions pre_emph: 0 | 1 | 2 | 3
      mask TypeOptions post_emph_r2: 0.18 | 0.19 | 0.2 | 0.39 | 0.63 | 0.82 | 1.07 | 1.32 | 1.6 | 1.65 | 1.94 | 2.21 | 2.52 | 2.76 | 3.08 | 3.41 | 3.77 | 3.97 | 4.36 | 4.73 | 5.16 | 5.47 | 5.93 | 6.38 | 6.89
      mask TypeOptions rxeqmix_r2: 0 | 1 | 2 | 3 | 4 | 5 | 6 | 7
      mask TypeOptions swing_r2: 110 | 210 | 310 | 400 | 480 | 570 | 660 | 740 | 810 | 880 | 940 | 990 | 1040 | 1080 | 1110 | 1130
      mask TypeOptions swing: 400 | 500 | 600 | 700 | 800
      mask Callback debug_en_all:
      | if strcmp(get_param(gcb, 'debug_en_all'), 'on')
      |     set_param(gcb, 'debug_dis_all', 'off')
      | end
      mask Callback debug_dis_all:
      | if strcmp(get_param(gcb, 'debug_dis_all'), 'on')
      |     set_param(gcb, 'debug_en_all', 'off')
      | end
      mask Callback txerrctr:
      | blk = gcb;
      | mask_visibilities = get_param(blk, 'MaskVisibilities');
      | mask_names = get_param(blk, 'MaskNames');
      | if strcmp(get_param(blk, 'txerrctr'), 'on')
      |     mask_visibilities{ismember(mask_names, 'txerrctr_len')} = 'on';
      | else
      |     mask_visibilities{ismember(mask_names, 'txerrctr_len')} = 'off';
      | end
      | set_param(blk, 'MaskVisibilities', mask_visibilities);
      mask TypeOptions txsnaplen: 0 - no snap | 256 | 512 | 1024 | 2048 | 4096 | 8192 | 16384
      mask Callback rxerrctr:
      | blk = gcb;
      | mask_visibilities = get_param(blk, 'MaskVisibilities');
      | mask_names = get_param(blk, 'MaskNames');
      | if strcmp(get_param(blk, 'rxerrctr'), 'on')
      |     mask_visibilities{ismember(mask_names, 'rxerrctr_len')} = 'on';
      | else
      |     mask_visibilities{ismember(mask_names, 'rxerrctr_len')} = 'off';
      | end
      | set_param(blk, 'MaskVisibilities', mask_visibilities);
      mask TypeOptions rxsnaplen: 0 - no snap | 256 | 512 | 1024 | 2048 | 4096 | 8192 | 16384
      mask DialogControl ParameterTabVar0 Prompt: Core
      mask DialogControl ParameterTabVar01 Prompt: Debug counters
      mask DialogControl Control2 Prompt: -------------------------------------
      mask DialogControl Control2_copy Prompt: -------------------------------------
  wires:
  Constant/1 -> onehundred_gbe/7(rx_ack)
  Slice3/1 -> [gbe_stat_rst]
  Slice2/1 -> [gbe_port]
  Slice1/1 -> [gbe_sw_en]
  Slice/1 -> [gbe_sw_rst]
  ctrl/1(in_reg) -> Slice/1, Slice1/1, Slice2/1, Slice3/1
  vld/1 -> Logical/1
  Logical/1 -> onehundred_gbe/3(tx_valid)
  dest_ip/1 -> onehundred_gbe/4(tx_dest_ip)
  eof/1 -> onehundred_gbe/6(tx_end_of_frame), Register/2
  data/1 -> onehundred_gbe/2(tx_data)
  [gbe_sw_rst] -> Delay/1
  Register/1 -> Logical/2
  [gbe_sw_en] -> Register/1
  Delay/1 -> onehundred_gbe/1(rst)
  Constant1/1 -> onehundred_gbe/8(rx_overrun_ack)
  [gbe_stat_rst] -> onehundred_gbe/9(debug_rst)
  byte_enable/1 -> onehundred_gbe/10(tx_byte_enable)
  dest_port/1 -> onehundred_gbe/5(tx_dest_port)
